simulink model "AFS_VD"  (R2016b)
settings: configuration reference "CodeGenConfigSet" (kept outside this file)
values from neighbouring files (symbols this model uses):
  AFS_dmAirSubsVal_MAP = Calibration.Parameter    [init_AFS_VD.m]
  AFS_dmAirSubsVal_MAPX = Calibration.Parameter    [init_AFS_VD.m]
  AFS_dmAirSubsVal_MAPY = Calibration.Parameter    [init_AFS_VD.m]
  AFS_dtAirThresHi_C = Calibration.Parameter    [init_AFS_VD.m]
  AFS_dtAirThresLo_C = Calibration.Parameter    [init_AFS_VD.m]
  AFS_facAirNrmPT1_C = Calibration.Parameter    [init_AFS_VD.m]
  AFS_facAirSubsEnvPCor_CUR = Calibration.Parameter    [init_AFS_VD.m]
  AFS_facAirSubsEnvPCor_CURX = Calibration.Parameter    [init_AFS_VD.m]
  AFS_facPlsCorBasEGRShOff_MAP = Calibration.Parameter    [init_AFS_VD.m]
  AFS_facPlsCorBasEGRShOff_MAPX = Calibration.Parameter    [init_AFS_VD.m]
  AFS_facPlsCorBasEGRShOff_MAPY = Calibration.Parameter    [init_AFS_VD.m]
  AFS_facPlsCorBasEOMQnt2_MAP = Calibration.Parameter    [init_AFS_VD.m]
  AFS_facPlsCorBasEOMQnt2_MAPX = Calibration.Parameter    [init_AFS_VD.m]
  AFS_facPlsCorBasEOMQnt2_MAPY = Calibration.Parameter    [init_AFS_VD.m]
  AFS_facSwtOnCor_C = Calibration.Parameter    [init_AFS_VD.m]
  AFS_MAIRCONV = int32(33333)    [init_AFS_VD.m]
  AFS_nAvrgThresHi_C = Calibration.Parameter    [init_AFS_VD.m]
  AFS_nAvrgThresLo_C = Calibration.Parameter    [init_AFS_VD.m]
  AFS_numAirTemp_C = Calibration.Parameter    [init_AFS_VD.m]
  AFS_numEngTemp_C = Calibration.Parameter    [init_AFS_VD.m]
  AFS_pAirThrLo_C = Calibration.Parameter    [init_AFS_VD.m]
  AFS_pBstThresHi_C = Calibration.Parameter    [init_AFS_VD.m]
  AFS_pBstThresLo_C = Calibration.Parameter    [init_AFS_VD.m]
  AFS_qRawOvrRunThresHi_C = Calibration.Parameter    [init_AFS_VD.m]
  AFS_qRawOvrRunThresLo_C = Calibration.Parameter    [init_AFS_VD.m]
  AFS_rAirThresIdlHi_C = Calibration.Parameter    [init_AFS_VD.m]
  AFS_rAirThresIdlLo_C = Calibration.Parameter    [init_AFS_VD.m]
  AFS_rAirThresLdHi_C = Calibration.Parameter    [init_AFS_VD.m]
  AFS_rAirThresLdLo_C = Calibration.Parameter    [init_AFS_VD.m]
  AFS_rAirThresOvrRunHi_C = Calibration.Parameter    [init_AFS_VD.m]
  AFS_rAirThresOvrRunLo_C = Calibration.Parameter    [init_AFS_VD.m]
  AFS_rEGRThresHi_C = Calibration.Parameter    [init_AFS_VD.m]
  AFS_rEGRThresLo_C = Calibration.Parameter    [init_AFS_VD.m]
  AFS_rTVAThrHi_C = Calibration.Parameter    [init_AFS_VD.m]
  AFS_rTVAThrLo_C = Calibration.Parameter    [init_AFS_VD.m]
  AFS_swtEnaPlsCor_C = Calibration.Parameter    [init_AFS_VD.m]
  AFS_swtPlausChkIdl_C = Calibration.Parameter    [init_AFS_VD.m]
  AFS_swtPlausChkLd_C = Calibration.Parameter    [init_AFS_VD.m]
  AFS_swtPlausChkOvrRun_C = Calibration.Parameter    [init_AFS_VD.m]
  AFS_swtSensInstVal_C = Calibration.Parameter    [init_AFS_VD.m]
  AFS_tAirThresHi_C = Calibration.Parameter    [init_AFS_VD.m]
  AFS_tAirThresLo_C = Calibration.Parameter    [init_AFS_VD.m]
  AFS_tEngThresHi_C = Calibration.Parameter    [init_AFS_VD.m]
  AFS_tEngThresLo_C = Calibration.Parameter    [init_AFS_VD.m]
  AFS_tiDlyEGRPPlSetyDrft_C = Calibration.Parameter    [init_AFS_VD.m]
  AFS_tiDlySwtOnCor_C = Calibration.Parameter    [init_AFS_VD.m]
  AFS_tiSetyDrftMaxDebDef_C = Calibration.Parameter    [init_AFS_VD.m]
  AFS_tiSetyDrftMaxDebOk_C = Calibration.Parameter    [init_AFS_VD.m]
  AFS_tiSetyDrftMinDebDef_C = Calibration.Parameter    [init_AFS_VD.m]
  AFS_tiSetyDrftMinDebOk_C = Calibration.Parameter    [init_AFS_VD.m]
  Epm_numCyl_C = Calibration.Parameter    [init_AFS_VD.m]
  SigTst_dmAFSVal_C = Calibration.Parameter    [init_AFS_VD.m]
  SigTst_mAirPerCyl_C = Calibration.Parameter    [init_AFS_VD.m]
  SigTst_swtAFSSubsVal_C = Calibration.Parameter    [init_AFS_VD.m]
  SigTst_swtAFSVal_C = Calibration.Parameter    [init_AFS_VD.m]
  SigTst_swtAirPerCyl_C = Calibration.Parameter    [init_AFS_VD.m]
undefined symbols (not defined in the file or in its folder): AFS_VD_DT, EngState_conv, Switch_conv
libraries: simulink x44, CXLib x10
settings Model: Creator=lenovo  LastModifiedBy=guanxiaoxing
settings ConfigSetRef: SourceLocation=Base Workspace

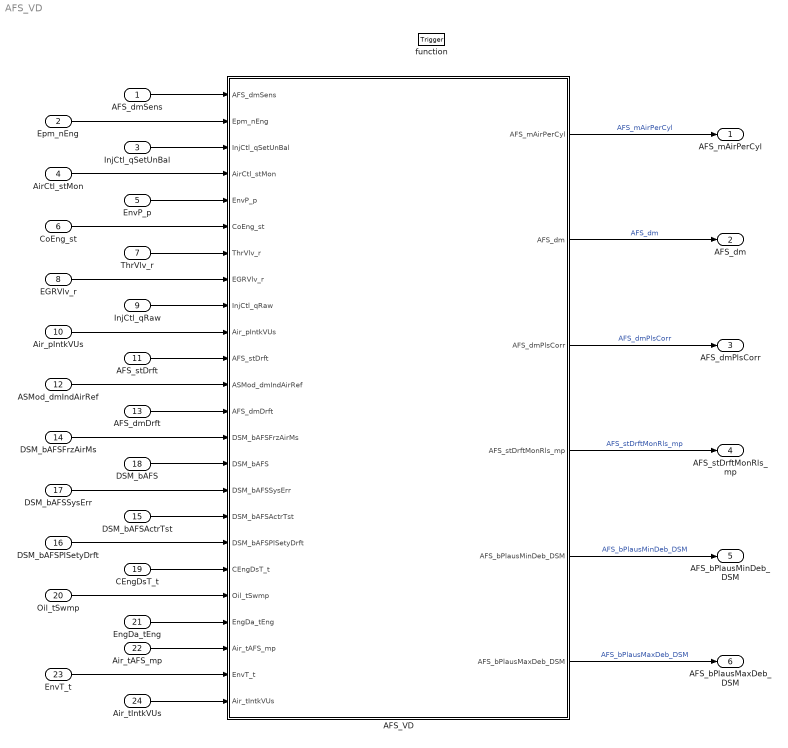
== system AFS_VD ==
  AFS_dmSens : Inport  Tag=kg/h  Description=Processed air mass flow signal of the HFM sensor  OutMin=-8192  OutMax=8191  OutDataTypeStr=AirMassPerTime
  Epm_nEng : Inport  Tag=rpm  Description=Engine speed  Port=2  OutMin=0  OutMax=6000  OutDataTypeStr=EngSpeed_rpm
  InjCtl_qSetUnBal : Inport  Tag=mg/hub  Description=Current injection quantity  Port=3  OutMin=-319  OutMax=319  OutDataTypeStr=FuelMass_mg_hub
  AirCtl_stMon : Inport  Description=status: shutdown case of the governor  Port=4  OutMin=0  OutMax=255  OutDataTypeStr=State_uint8
  EnvP_p : Inport  Tag=kPa  Description=Barometric pressure  Port=5  OutMin=0  OutMax=3276  OutDataTypeStr=AirPressure_kPa
  CoEng_st : Inport  Description=Engine coordinator state  Port=6  OutDataTypeStr=Enum: EngState_conv
  ThrVlv_r : Inport  Tag=%  Description=Commanded value from application SW  Port=7  OutMin=-100  OutMax=100  OutDataTypeStr=Prc_100_rate
  EGRVlv_r : Inport  Tag=%  Description=Commanded value from application SW  Port=8  OutMin=-100  OutMax=100  OutDataTypeStr=Prc_100_rate
  InjCtl_qRaw : Inport  Tag=mg/hub  Description=Raw value of injection mass  Port=9  OutMin=-319  OutMax=319  OutDataTypeStr=FuelMass_mg_hub
  Air_pIntkVUs : Inport  Tag=kPa  Description=Intake valve upstream pressure  Port=10  OutMin=0  OutMax=1200  OutDataTypeStr=AirPressure_kPa
  AFS_stDrft : Inport  Description=Status of drift compensation  Port=11  OutMin=0  OutMax=255  OutDataTypeStr=State_uint8
  ASMod_dmIndAirRef : Inport  Tag=kg/h  Description=Reference of gas mass flow into the engine while exhaust-gas recirculation is closed  Port=12  OutMin=-8192  OutMax=8191  OutDataTypeStr=AirMassPerTime
  AFS_dmDrft : Inport  Tag=kg/h  Description=Compensated Air mass value for the drift  Port=13  OutMin=-8192  OutMax=8191  OutDataTypeStr=AirMassPerTime
  DSM_bAFSFrzAirMs : Inport  Description=Function identifier to freeze the air mass value in case of temporary SRC errors  Port=14  OutMin=0  OutMax=1  OutDataTypeStr=boolean
  DSM_bAFSActrTst : Inport  Description=Function identifier to inhibit checks if remote tester is active for any of the actuators for swirl valve,throttle valve, turbo charger, EGR valve  Port=15  OutMin=0  OutMax=1  OutDataTypeStr=boolean
  DSM_bAFSPlSetyDrft : Inport  Description=Function identifier to inhibit the sensitivity drift check  Port=16  OutMin=0  OutMax=1  OutDataTypeStr=boolean
  DSM_bAFSSysErr : Inport  Description=Function identifier to inhibit the sensitivity drift check  Port=17  OutMin=0  OutMax=1  OutDataTypeStr=boolean
  DSM_bAFS : Inport  Description=Function identifier for switch-over value calculation  Port=18  OutMin=0  OutMax=1  OutDataTypeStr=boolean
  CEngDsT_t : Inport  Tag=deg  Description=engine coolant temperature after filter  Port=19  OutMin=-200  OutMax=200  OutDataTypeStr=Temp_deg
  Oil_tSwmp : Inport  Tag=deg  Description=Oil temperature in oil sump  Port=20  OutMin=-50  OutMax=200  OutDataTypeStr=Temp_deg
  EngDa_tEng : Inport  Tag=deg  Description=Engine temperature  Port=21  OutMin=-1000  OutMax=1000  OutDataTypeStr=Temp_deg
  Air_tAFS_mp : Inport  Tag=deg  Description=Induction air temperature at the HFM  Port=22  OutMin=-200  OutMax=200  OutDataTypeStr=Temp_deg
  EnvT_t : Inport  Tag=deg  Description=Environmental temperature  Port=23  OutMin=-200  OutMax=200  OutDataTypeStr=Temp_deg
  Air_tIntkVUs : Inport  Tag=deg  Description=Intake air temperature upstream of the inlet valve  Port=24  OutMin=-200  OutMax=200  OutDataTypeStr=Temp_deg
  function : TriggerPort  TriggerType=function-call  VariantControl=Variant
  AFS_VD : Subsystem
  AFS_mAirPerCyl : Outport  Tag=mg/hub  Description=Air mass per cylinder  OutMin=0  OutMax=16383  OutDataTypeStr=AirMass_mg_hub
  AFS_dm : Outport  Tag=kg/h  Description=Total air mass flow into the engine  Port=2  OutMin=-8192  OutMax=8191  OutDataTypeStr=AirMassPerTime
  AFS_dmPlsCorr : Outport  Tag=kg/h  Description=Pulsation corrected air mass.  Port=3  OutMin=-8192  OutMax=8191  OutDataTypeStr=AirMassPerTime
  AFS_stDrftMonRls_mp : Outport  Description=Status of monitoring conditions for the sensitivity drift test  Port=4  OutMin=0  OutMax=1  OutDataTypeStr=boolean
  AFS_bPlausMinDeb_DSM : Outport  Description=fault flag for plausibility check of Min error  Port=5  OutMin=0  OutMax=1  OutDataTypeStr=boolean
  AFS_bPlausMaxDeb_DSM : Outport  Description=fault flag for plausibility check of Max error  Port=6  OutMin=0  OutMax=1  OutDataTypeStr=boolean
  wires:
  AFS_VD/1(AFS_mAirPerCyl) -> AFS_mAirPerCyl/1  "AFS_mAirPerCyl"
  AFS_VD/2(AFS_dm) -> AFS_dm/1  "AFS_dm"
  AFS_VD/3(AFS_dmPlsCorr) -> AFS_dmPlsCorr/1  "AFS_dmPlsCorr"
  AFS_VD/4(AFS_stDrftMonRls_mp) -> AFS_stDrftMonRls_mp/1  "AFS_stDrftMonRls_mp"
  AFS_VD/5(AFS_bPlausMinDeb_DSM) -> AFS_bPlausMinDeb_DSM/1  "AFS_bPlausMinDeb_DSM"
  AFS_VD/6(AFS_bPlausMaxDeb_DSM) -> AFS_bPlausMaxDeb_DSM/1  "AFS_bPlausMaxDeb_DSM"
  AFS_dmSens/1 -> AFS_VD/1(AFS_dmSens)
  Epm_nEng/1 -> AFS_VD/2(Epm_nEng)
  InjCtl_qSetUnBal/1 -> AFS_VD/3(InjCtl_qSetUnBal)
  AirCtl_stMon/1 -> AFS_VD/4(AirCtl_stMon)
  EnvP_p/1 -> AFS_VD/5(EnvP_p)
  CoEng_st/1 -> AFS_VD/6(CoEng_st)
  ThrVlv_r/1 -> AFS_VD/7(ThrVlv_r)
  EGRVlv_r/1 -> AFS_VD/8(EGRVlv_r)
  InjCtl_qRaw/1 -> AFS_VD/9(InjCtl_qRaw)
  Air_pIntkVUs/1 -> AFS_VD/10(Air_pIntkVUs)
  AFS_stDrft/1 -> AFS_VD/11(AFS_stDrft)
  ASMod_dmIndAirRef/1 -> AFS_VD/12(ASMod_dmIndAirRef)
  AFS_dmDrft/1 -> AFS_VD/13(AFS_dmDrft)
  DSM_bAFSFrzAirMs/1 -> AFS_VD/14(DSM_bAFSFrzAirMs)
  DSM_bAFS/1 -> AFS_VD/15(DSM_bAFS)
  DSM_bAFSActrTst/1 -> AFS_VD/17(DSM_bAFSActrTst)
  DSM_bAFSSysErr/1 -> AFS_VD/16(DSM_bAFSSysErr)
  DSM_bAFSPlSetyDrft/1 -> AFS_VD/18(DSM_bAFSPlSetyDrft)
  CEngDsT_t/1 -> AFS_VD/19(CEngDsT_t)
  Oil_tSwmp/1 -> AFS_VD/20(Oil_tSwmp)
  EngDa_tEng/1 -> AFS_VD/21(EngDa_tEng)
  Air_tAFS_mp/1 -> AFS_VD/22(Air_tAFS_mp)
  EnvT_t/1 -> AFS_VD/23(EnvT_t)
  Air_tIntkVUs/1 -> AFS_VD/24(Air_tIntkVUs)

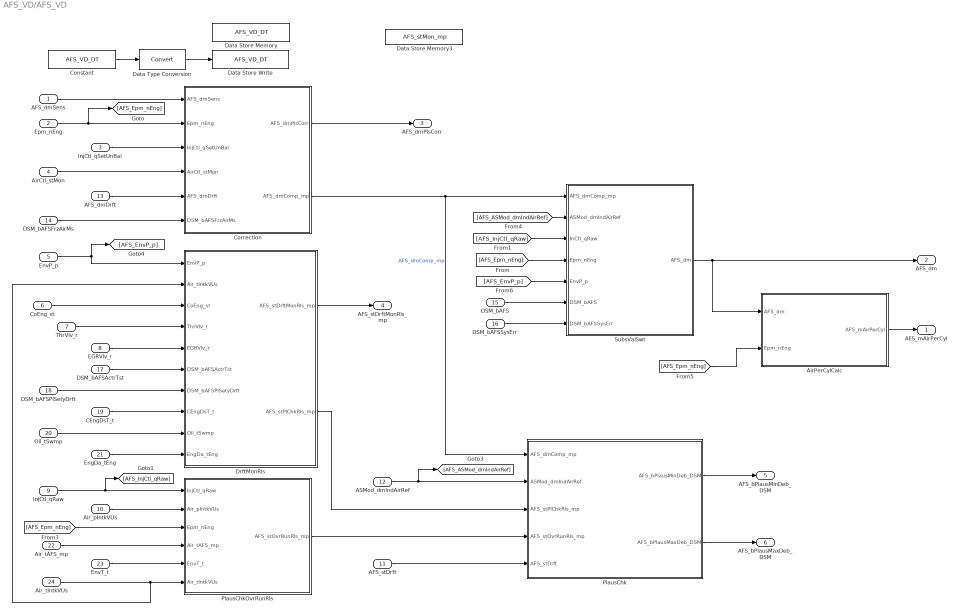
== system AFS_VD/AFS_VD ==
  AFS_dmSens : Inport
  Epm_nEng : Inport  Port=2
  InjCtl_qSetUnBal : Inport  Port=3
  AirCtl_stMon : Inport  Port=4
  EnvP_p : Inport  Port=5
  CoEng_st : Inport  Port=6
  ThrVlv_r : Inport  Port=7
  EGRVlv_r : Inport  Port=8
  InjCtl_qRaw : Inport  Port=9
  Air_pIntkVUs : Inport  Port=10
  AFS_stDrft : Inport  Port=11
  ASMod_dmIndAirRef : Inport  Port=12
  AFS_dmDrft : Inport  Port=13
  DSM_bAFSFrzAirMs : Inport  Port=14
  DSM_bAFS : Inport  Port=15
  DSM_bAFSSysErr : Inport  Port=16
  DSM_bAFSActrTst : Inport  Port=17
  DSM_bAFSPlSetyDrft : Inport  Port=18
  CEngDsT_t : Inport  Port=19
  Oil_tSwmp : Inport  Port=20
  EngDa_tEng : Inport  Port=21
  Air_tAFS_mp : Inport  Port=22
  EnvT_t : Inport  Port=23
  Air_tIntkVUs : Inport  Port=24
  AirPerCylCalc : Subsystem
  Constant : Constant  Value=AFS_VD_DT
  Correction : Subsystem
  Data Store Memory : DataStoreMemory  DataStoreName=AFS_VD_DT  ReadBeforeWriteMsg=warning  WriteAfterWriteMsg=warning  WriteAfterReadMsg=warning  ShowAdditionalParam=off
  Data Store Memory3 : DataStoreMemory  DataStoreName=AFS_stMon_mp  ReadBeforeWriteMsg=warning  WriteAfterWriteMsg=warning  WriteAfterReadMsg=warning  ShowAdditionalParam=off  StateMustResolveToSignalObject=on
  Data Store Write : DataStoreWrite  DataStoreName=AFS_VD_DT
  Data Type Conversion : DataTypeConversion
  DrftMonRls : Subsystem
  PlausChk : Subsystem
  PlausChkOvrRunRls : Subsystem
  SubsValSwt : Subsystem
  AFS_mAirPerCyl : Outport
  AFS_dm : Outport  Port=2
  AFS_dmPlsCorr : Outport  Port=3
  AFS_stDrftMonRls_mp : Outport  Port=4
  AFS_bPlausMinDeb_DSM : Outport  Port=5
  AFS_bPlausMaxDeb_DSM : Outport  Port=6
  wires:
  Epm_nEng/1 -> [AFS_Epm_nEng], Correction/2(Epm_nEng)
  InjCtl_qRaw/1 -> PlausChkOvrRunRls/1(InjCtl_qRaw), [AFS_InjCtl_qRaw]
  Air_pIntkVUs/1 -> PlausChkOvrRunRls/2(Air_pIntkVUs)
  DrftMonRls/2(AFS_stPlChkRls_mp) -> PlausChk/3(AFS_stPlChkRls_mp)
  DrftMonRls/1(AFS_stDrftMonRls_mp) -> AFS_stDrftMonRls_mp/1
  AirPerCylCalc/1(AFS_mAirPerCyl) -> AFS_mAirPerCyl/1
  [AFS_Epm_nEng] -> AirPerCylCalc/2(Epm_nEng)
  Air_tIntkVUs/1 -> DrftMonRls/2(Air_tIntkVUs), PlausChkOvrRunRls/6(Air_tIntkVUs)
  CoEng_st/1 -> DrftMonRls/3(CoEng_st)
  ThrVlv_r/1 -> DrftMonRls/4(ThrVlv_r)
  EGRVlv_r/1 -> DrftMonRls/5(EGRVlv_r)
  AFS_stDrft/1 -> PlausChk/5(AFS_stDrft)
  ASMod_dmIndAirRef/1 -> PlausChk/2(ASMod_dmIndAirRef), [AFS_ASMod_dmIndAirRef]
  PlausChkOvrRunRls/1(AFS_stOvrRunRls_mp) -> PlausChk/4(AFS_stOvrRunRls_mp)
  [AFS_Epm_nEng] -> PlausChkOvrRunRls/3(Epm_nEng)
  SubsValSwt/1(AFS_dm) -> AFS_dm/1, AirPerCylCalc/1(AFS_dm)
  EnvP_p/1 -> [AFS_EnvP_p], DrftMonRls/1(EnvP_p)
  [AFS_InjCtl_qRaw] -> SubsValSwt/3(InCtl_qRaw)
  [AFS_Epm_nEng] -> SubsValSwt/4(Epm_nEng)
  [AFS_ASMod_dmIndAirRef] -> SubsValSwt/2(ASMod_dmIndAirRef)
  [AFS_EnvP_p] -> SubsValSwt/5(EnvP_p)
  Constant/1 -> Data Type Conversion/1
  Correction/2(AFS_dmComp_mp) -> SubsValSwt/1(AFS_dmComp_mp), PlausChk/1(AFS_dmComp_mp)  "AFS_dmComp_mp"
  AFS_dmSens/1 -> Correction/1(AFS_dmSens)
  InjCtl_qSetUnBal/1 -> Correction/3(InjCtl_qSetUnBal)
  AirCtl_stMon/1 -> Correction/4(AirCtl_stMon)
  AFS_dmDrft/1 -> Correction/5(AFS_dmDrft)
  DSM_bAFSFrzAirMs/1 -> Correction/6(DSM_bAFSFrzAirMs)
  Correction/1(AFS_dmPlsCorr) -> AFS_dmPlsCorr/1
  DSM_bAFS/1 -> SubsValSwt/6(DSM_bAFS)
  DSM_bAFSSysErr/1 -> SubsValSwt/7(DSM_bAFSSysErr)
  DSM_bAFSActrTst/1 -> DrftMonRls/6(DSM_bAFSActrTst)
  DSM_bAFSPlSetyDrft/1 -> DrftMonRls/7(DSM_bAFSPlSetyDrft)
  CEngDsT_t/1 -> DrftMonRls/8(CEngDsT_t)
  Oil_tSwmp/1 -> DrftMonRls/9(Oil_tSwmp)
  EngDa_tEng/1 -> DrftMonRls/10(EngDa_tEng)
  Air_tAFS_mp/1 -> PlausChkOvrRunRls/4(Air_tAFS_mp)
  EnvT_t/1 -> PlausChkOvrRunRls/5(EnvT_t)
  PlausChk/1(AFS_bPlausMinDeb_DSM) -> AFS_bPlausMinDeb_DSM/1
  PlausChk/2(AFS_bPlausMaxDeb_DSM) -> AFS_bPlausMaxDeb_DSM/1
  Data Type Conversion/1 -> Data Store Write/1

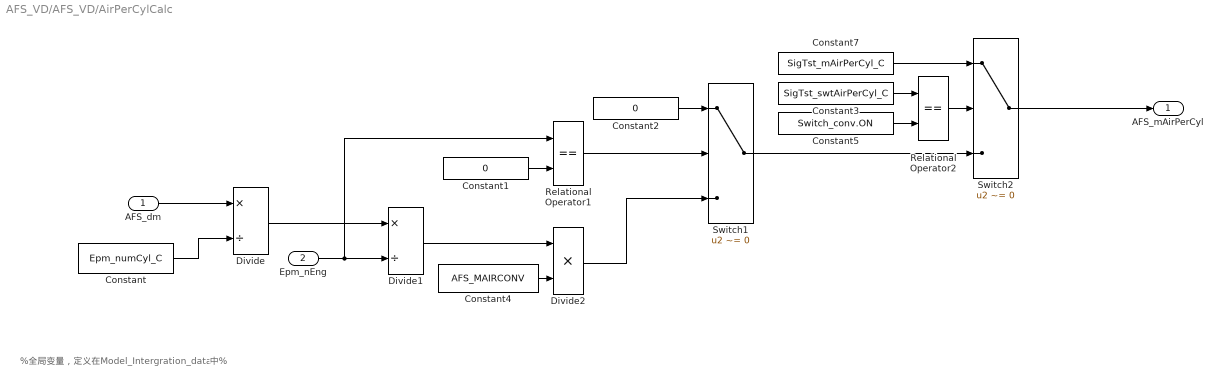
== system AFS_VD/AFS_VD/AirPerCylCalc ==
  note: %全局变量，定义在Model_Intergration_data中%
  AFS_dm : Inport
  Epm_nEng : Inport  Port=2
  Constant : Constant  Value=Epm_numCyl_C
  Constant1 : Constant  Value=0  OutDataTypeStr=EngSpeed_rpm
  Constant2 : Constant  Value=0  OutDataTypeStr=AirMass_mg_hub
  Constant3 : Constant  Value=SigTst_swtAirPerCyl_C
  Constant4 : Constant  Value=AFS_MAIRCONV
  Constant5 : Constant  Value=Switch_conv.ON
  Constant7 : Constant  Value=SigTst_mAirPerCyl_C
  Divide : Product  Inputs=*/  OutDataTypeStr=Inherit: Inherit via back propagation  SaturateOnIntegerOverflow=on
  Divide1 : Product  Inputs=*/  OutDataTypeStr=fixdt(1,32,16)  SaturateOnIntegerOverflow=on
  Divide2 : Product  Inputs=**  OutDataTypeStr=Inherit: Inherit via back propagation  SaturateOnIntegerOverflow=on
  Relational Operator1 : RelationalOperator  Operator===  OutDataTypeStr=boolean  RndMeth=Nearest  InputSameDT=on
  Relational Operator2 : RelationalOperator  Operator===  OutDataTypeStr=boolean  RndMeth=Nearest  InputSameDT=on
  Switch1 : Switch  Criteria=u2 ~= 0  OutDataTypeStr=Inherit: Inherit via back propagation  SaturateOnIntegerOverflow=on  InputSameDT=on
  Switch2 : Switch  Criteria=u2 ~= 0  OutDataTypeStr=Inherit: Inherit via back propagation  SaturateOnIntegerOverflow=on  InputSameDT=on
  AFS_mAirPerCyl : Outport
  wires:
  Constant5/1 -> Relational Operator2/2
  Switch1/1 -> Switch2/3
  Constant7/1 -> Switch2/1
  Relational Operator2/1 -> Switch2/2
  Constant3/1 -> Relational Operator2/1
  Constant2/1 -> Switch1/1
  Divide2/1 -> Switch1/3
  AFS_dm/1 -> Divide/1
  Relational Operator1/1 -> Switch1/2
  Constant1/1 -> Relational Operator1/2
  Epm_nEng/1 -> Divide1/2, Relational Operator1/1
  Constant4/1 -> Divide2/2
  Divide/1 -> Divide1/1
  Divide1/1 -> Divide2/1
  Switch2/1 -> AFS_mAirPerCyl/1
  Constant/1 -> Divide/2

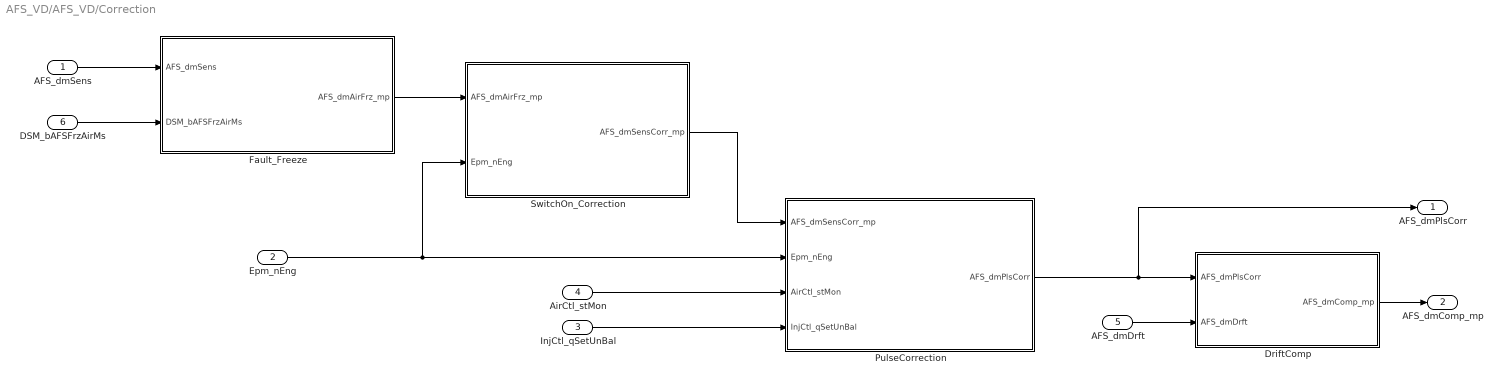
== system AFS_VD/AFS_VD/Correction ==
  AFS_dmSens : Inport
  Epm_nEng : Inport  Port=2
  InjCtl_qSetUnBal : Inport  Port=3
  AirCtl_stMon : Inport  Port=4
  AFS_dmDrft : Inport  Port=5
  DSM_bAFSFrzAirMs : Inport  Port=6
  DriftComp : Subsystem
  Fault_Freeze : Subsystem
  PulseCorrection : Subsystem
  SwitchOn_Correction : Subsystem
  AFS_dmPlsCorr : Outport
  AFS_dmComp_mp : Outport  Port=2
  wires:
  PulseCorrection/1(AFS_dmPlsCorr) -> DriftComp/1(AFS_dmPlsCorr), AFS_dmPlsCorr/1
  InjCtl_qSetUnBal/1 -> PulseCorrection/4(InjCtl_qSetUnBal)
  AirCtl_stMon/1 -> PulseCorrection/3(AirCtl_stMon)
  SwitchOn_Correction/1(AFS_dmSensCorr_mp) -> PulseCorrection/1(AFS_dmSensCorr_mp)
  Fault_Freeze/1(AFS_dmAirFrz_mp) -> SwitchOn_Correction/1(AFS_dmAirFrz_mp)
  Epm_nEng/1 -> SwitchOn_Correction/2(Epm_nEng), PulseCorrection/2(Epm_nEng)
  AFS_dmSens/1 -> Fault_Freeze/1(AFS_dmSens)
  DSM_bAFSFrzAirMs/1 -> Fault_Freeze/2(DSM_bAFSFrzAirMs)
  AFS_dmDrft/1 -> DriftComp/2(AFS_dmDrft)
  DriftComp/1(AFS_dmComp_mp) -> AFS_dmComp_mp/1

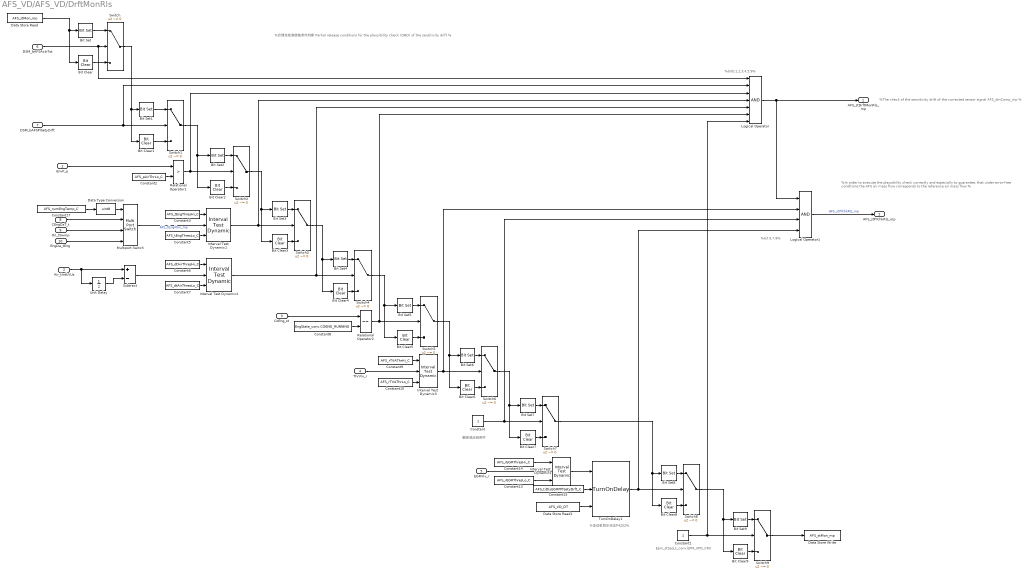
== system AFS_VD/AFS_VD/DrftMonRls ==
  note: Epm_stSpd_t_conv.EPM_SPD_CRS
  note: 删掉涡流阀条件
  note: %发动机同步状态P4252%
  note: %bit0,1,2,3,4,5,9%
  note: %bit 6,7,8%
  note: %The check of the sensitivity drift of the corrected sensor signal AFS_dmComp_mp %
  note: %In order to execute the plausibility check correctly and especially to guarantee, that under error-free conditions the AFS air mass flow corresponds
      | to the reference air mass flow %
  note: %合理性检测使能条件判断
      | Partial release conditions for the plausibility check (OBD) of the sensitivity drift %
  EnvP_p : Inport
  Air_tIntkVUs : Inport  Port=2
  CoEng_st : Inport  Port=3
  ThrVlv_r : Inport  Port=4
  EGRVlv_r : Inport  Port=5
  DSM_bAFSActrTst : Inport  Port=6
  DSM_bAFSPlSetyDrft : Inport  Port=7
  CEngDsT_t : Inport  Port=8
  Oil_tSwmp : Inport  Port=9
  EngDa_tEng : Inport  Port=10
  Bit Clear : simulink/Logic and Bit Operations/Bit Clear  iBit=0
  Bit Clear1 : simulink/Logic and Bit Operations/Bit Clear  iBit=1
  Bit Clear2 : simulink/Logic and Bit Operations/Bit Clear  iBit=2
  Bit Clear3 : simulink/Logic and Bit Operations/Bit Clear  iBit=3
  Bit Clear4 : simulink/Logic and Bit Operations/Bit Clear  iBit=4
  Bit Clear5 : simulink/Logic and Bit Operations/Bit Clear  iBit=5
  Bit Clear6 : simulink/Logic and Bit Operations/Bit Clear  iBit=6
  Bit Clear7 : simulink/Logic and Bit Operations/Bit Clear  iBit=7
  Bit Clear8 : simulink/Logic and Bit Operations/Bit Clear  iBit=8
  Bit Clear9 : simulink/Logic and Bit Operations/Bit Clear  iBit=9
  Bit Set : simulink/Logic and Bit Operations/Bit Set  iBit=0
  Bit Set1 : simulink/Logic and Bit Operations/Bit Set  iBit=1
  Bit Set2 : simulink/Logic and Bit Operations/Bit Set  iBit=2
  Bit Set3 : simulink/Logic and Bit Operations/Bit Set  iBit=3
  Bit Set4 : simulink/Logic and Bit Operations/Bit Set  iBit=4
  Bit Set5 : simulink/Logic and Bit Operations/Bit Set  iBit=5
  Bit Set6 : simulink/Logic and Bit Operations/Bit Set  iBit=6
  Bit Set7 : simulink/Logic and Bit Operations/Bit Set  iBit=7
  Bit Set8 : simulink/Logic and Bit Operations/Bit Set  iBit=8
  Bit Set9 : simulink/Logic and Bit Operations/Bit Set  iBit=9
  Constant : Constant  OutDataTypeStr=boolean
  Constant1 : Constant  OutDataTypeStr=boolean
  Constant10 : Constant  Value=AFS_rTVAThrLo_C
  Constant13 : Constant  Value=AFS_rEGRThresLo_C
  Constant14 : Constant  Value=AFS_rEGRThresHi_C
  Constant15 : Constant  Value=AFS_tiDlyEGRPPlSetyDrft_C
  Constant17 : Constant  Value=AFS_numEngTemp_C
  Constant2 : Constant  Value=AFS_pAirThrLo_C
  Constant3 : Constant  Value=AFS_tEngThresHi_C
  Constant5 : Constant  Value=AFS_tEngThresLo_C
  Constant6 : Constant  Value=AFS_dtAirThresHi_C
  Constant7 : Constant  Value=AFS_dtAirThresLo_C
  Constant8 : Constant  Value=EngState_conv.COENG_RUNNING
  Constant9 : Constant  Value=AFS_rTVAThrHi_C
  Data Store Read : DataStoreRead  DataStoreName=AFS_stMon_mp
  Data Store Read1 : DataStoreRead  DataStoreName=AFS_VD_DT
  Data Store Write : DataStoreWrite  DataStoreName=AFS_stMon_mp
  Data Type Conversion : DataTypeConversion  OutDataTypeStr=uint8
  Interval Test Dynamic{1..3,5} (4 alike) : simulink/Logic and Bit Operations/Interval Test Dynamic  IntervalClosedRight=on  IntervalClosedLeft=on  OutDataTypeStr=boolean
  Logical Operator : Logic  Inputs=7  AllPortsSameDT=off  OutDataTypeStr=boolean
  Logical Operator1 : Logic  Inputs=4  AllPortsSameDT=off  OutDataTypeStr=boolean
  Multiport Switch : MultiPortSwitch  DataPortOrder=Zero-based contiguous
  Relational Operator1 : RelationalOperator  Operator=>  OutDataTypeStr=boolean  RndMeth=Nearest  InputSameDT=on
  Relational Operator2 : RelationalOperator  Operator===  OutDataTypeStr=boolean  RndMeth=Nearest  InputSameDT=on
  Subtract : Sum  Inputs=+-  OutDataTypeStr=Temp_deg_s
  Switch{,1..9} (10 alike) : Switch  Criteria=u2 ~= 0  OutDataTypeStr=Inherit: Inherit via back propagation  SaturateOnIntegerOverflow=on  InputSameDT=on
  TurnOnDelay1 : CXLib/TurnOnDelay
  Unit Delay : UnitDelay  SampleTime=-1
  AFS_stDrftMonRls_mp : Outport
  AFS_stPlChkRls_mp : Outport  Port=2
  wires:
  Multiport Switch/1 -> Interval Test Dynamic1/2  "AFS_tEngMon_mp"
  Constant17/1 -> Data Type Conversion/1
  Switch9/1 -> Data Store Write/1
  TurnOnDelay1/1 -> Logical Operator1/4, Switch8/2
  Interval Test Dynamic5/1 -> TurnOnDelay1/1
  Constant15/1 -> TurnOnDelay1/2
  Switch7/1 -> Bit Set8/1, Bit Clear8/1
  Data Store Read1/1 -> TurnOnDelay1/3
  Bit Clear8/1 -> Switch8/3
  Constant13/1 -> Interval Test Dynamic5/3
  Constant14/1 -> Interval Test Dynamic5/1
  EGRVlv_r/1 -> Interval Test Dynamic5/2
  Bit Set8/1 -> Switch8/1
  Interval Test Dynamic3/1 -> Switch6/2, Logical Operator1/2
  Switch6/1 -> Bit Clear7/1, Bit Set7/1
  Bit Set7/1 -> Switch7/1
  Constant10/1 -> Interval Test Dynamic3/3
  Constant9/1 -> Interval Test Dynamic3/1
  Bit Clear7/1 -> Switch7/3
  Bit Set6/1 -> Switch6/1
  Bit Clear6/1 -> Switch6/3
  Bit Set5/1 -> Switch5/1
  Switch5/1 -> Bit Set6/1, Bit Clear6/1
  ThrVlv_r/1 -> Interval Test Dynamic3/2
  Switch1/1 -> Bit Set2/1, Bit Clear2/1
  Constant3/1 -> Interval Test Dynamic1/1
  Relational Operator1/1 -> Switch2/2, Logical Operator/3
  Bit Clear1/1 -> Switch1/3
  Switch2/1 -> Bit Set3/1, Bit Clear3/1
  Bit Set3/1 -> Switch3/1
  Interval Test Dynamic1/1 -> Switch3/2, Logical Operator/4
  Bit Clear3/1 -> Switch3/3
  Switch3/1 -> Bit Clear4/1, Bit Set4/1
  Bit Clear4/1 -> Switch4/3
  Bit Set4/1 -> Switch4/1
  Interval Test Dynamic2/1 -> Switch4/2, Logical Operator/5
  Constant7/1 -> Interval Test Dynamic2/3
  Constant6/1 -> Interval Test Dynamic2/1
  Constant2/1 -> Relational Operator1/2
  Constant5/1 -> Interval Test Dynamic1/3
  Switch4/1 -> Bit Clear5/1, Bit Set5/1
  Constant8/1 -> Relational Operator2/2
  Relational Operator2/1 -> Switch5/2, Logical Operator/6
  Bit Clear5/1 -> Switch5/3
  Switch/1 -> Bit Clear1/1, Bit Set1/1
  CoEng_st/1 -> Relational Operator2/1
  Switch8/1 -> Bit Clear9/1, Bit Set9/1
  Bit Clear9/1 -> Switch9/3
  Bit Set9/1 -> Switch9/1
  Logical Operator1/1 -> AFS_stPlChkRls_mp/1  "AFS_stPlChkRls_mp"
  Logical Operator/1 -> Logical Operator1/1, AFS_stDrftMonRls_mp/1
  Bit Set/1 -> Switch/1
  DSM_bAFSActrTst/1 -> Switch/2, Logical Operator/1
  EnvP_p/1 -> Relational Operator1/1
  Bit Clear/1 -> Switch/3
  Data Store Read/1 -> Bit Clear/1, Bit Set/1
  Bit Set1/1 -> Switch1/1
  DSM_bAFSPlSetyDrft/1 -> Switch1/2, Logical Operator/2
  Bit Clear2/1 -> Switch2/3
  Bit Set2/1 -> Switch2/1
  CEngDsT_t/1 -> Multiport Switch/2
  Oil_tSwmp/1 -> Multiport Switch/3
  EngDa_tEng/1 -> Multiport Switch/4
  Data Type Conversion/1 -> Multiport Switch/1
  Air_tIntkVUs/1 -> Unit Delay/1, Subtract/1
  Subtract/1 -> Interval Test Dynamic2/2
  Unit Delay/1 -> Subtract/2
  Constant/1 -> Logical Operator1/3, Switch7/2
  Constant1/1 -> Logical Operator/7, Switch9/2

== system AFS_VD/AFS_VD/PlausChk ==
  AFS_dmComp_mp : Inport
  ASMod_dmIndAirRef : Inport  Port=2
  AFS_stPlChkRls_mp : Inport  Port=3
  AFS_stOvrRunRls_mp : Inport  Port=4
  AFS_stDrft : Inport  Port=5
  Detect : Subsystem
  Monitor_Fault : Subsystem
  AFS_bPlausMinDeb_DSM : Outport
  AFS_bPlausMaxDeb_DSM : Outport  Port=2
  wires:
  AFS_stDrft/1 -> Detect/1(AFS_stDrft)
  AFS_dmComp_mp/1 -> Detect/2(AFS_dmComp_mp)
  ASMod_dmIndAirRef/1 -> Detect/3(ASMod_dmIndAirRef)
  AFS_stPlChkRls_mp/1 -> Monitor_Fault/1(AFS_stPlChkRls_mp)
  AFS_stOvrRunRls_mp/1 -> Monitor_Fault/2(AFS_stOvrRunRls_mp)
  Detect/1(stLoadRls) -> Monitor_Fault/3(stLoadRls)
  Detect/2(stIdlRls) -> Monitor_Fault/4(stIdlRls)
  Detect/3(stPlausMin) -> Monitor_Fault/5(stPlausMin)
  Detect/4(stPlausMax) -> Monitor_Fault/6(stPlausMax)
  Monitor_Fault/2(AFS_bPlausMaxDeb_DSM) -> AFS_bPlausMaxDeb_DSM/1
  Monitor_Fault/1(AFS_bPlausMinDeb_DSM) -> AFS_bPlausMinDeb_DSM/1

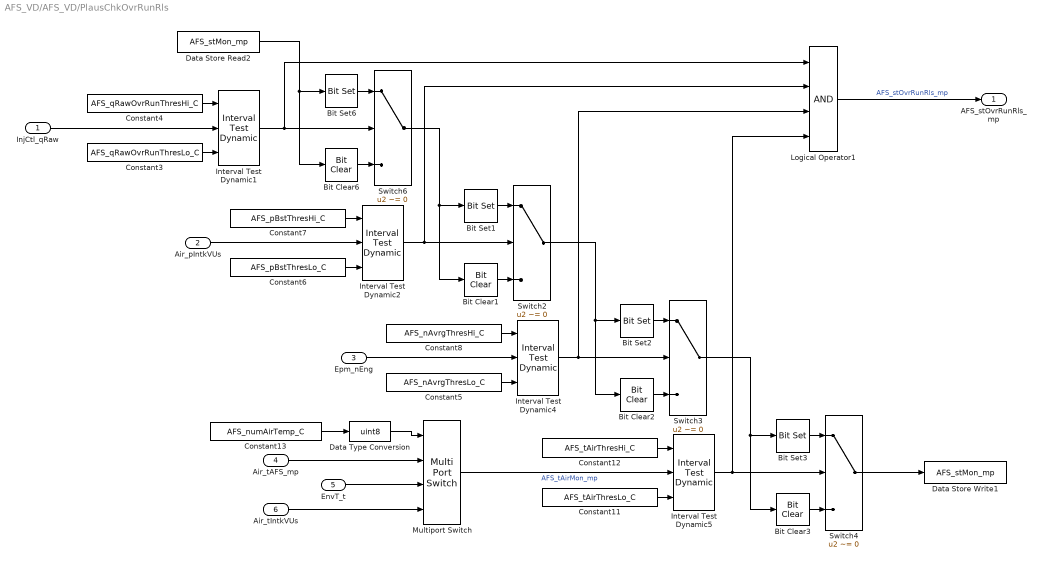
== system AFS_VD/AFS_VD/PlausChkOvrRunRls ==
  InjCtl_qRaw : Inport
  Air_pIntkVUs : Inport  Port=2
  Epm_nEng : Inport  Port=3
  Air_tAFS_mp : Inport  Port=4
  EnvT_t : Inport  Port=5
  Air_tIntkVUs : Inport  Port=6
  Bit Clear1 : simulink/Logic and Bit Operations/Bit Clear  iBit=16
  Bit Clear2 : simulink/Logic and Bit Operations/Bit Clear  iBit=17
  Bit Clear3 : simulink/Logic and Bit Operations/Bit Clear  iBit=18
  Bit Clear6 : simulink/Logic and Bit Operations/Bit Clear  iBit=15
  Bit Set1 : simulink/Logic and Bit Operations/Bit Set  iBit=16
  Bit Set2 : simulink/Logic and Bit Operations/Bit Set  iBit=17
  Bit Set3 : simulink/Logic and Bit Operations/Bit Set  iBit=18
  Bit Set6 : simulink/Logic and Bit Operations/Bit Set  iBit=15
  Constant11 : Constant  Value=AFS_tAirThresLo_C
  Constant12 : Constant  Value=AFS_tAirThresHi_C
  Constant13 : Constant  Value=AFS_numAirTemp_C
  Constant3 : Constant  Value=AFS_qRawOvrRunThresLo_C
  Constant4 : Constant  Value=AFS_qRawOvrRunThresHi_C
  Constant5 : Constant  Value=AFS_nAvrgThresLo_C
  Constant6 : Constant  Value=AFS_pBstThresLo_C
  Constant7 : Constant  Value=AFS_pBstThresHi_C
  Constant8 : Constant  Value=AFS_nAvrgThresHi_C
  Data Store Read2 : DataStoreRead  DataStoreName=AFS_stMon_mp
  Data Store Write1 : DataStoreWrite  DataStoreName=AFS_stMon_mp
  Data Type Conversion : DataTypeConversion  OutDataTypeStr=uint8
  Interval Test Dynamic{1..2,4..5} (4 alike) : simulink/Logic and Bit Operations/Interval Test Dynamic  IntervalClosedRight=on  IntervalClosedLeft=on  OutDataTypeStr=boolean
  Logical Operator1 : Logic  Inputs=4  AllPortsSameDT=off  OutDataTypeStr=boolean
  Multiport Switch : MultiPortSwitch  DataPortOrder=Zero-based contiguous
  Switch{2..4,6} (4 alike) : Switch  Criteria=u2 ~= 0  OutDataTypeStr=Inherit: Inherit via back propagation  SaturateOnIntegerOverflow=on  InputSameDT=on
  AFS_stOvrRunRls_mp : Outport
  wires:
  Multiport Switch/1 -> Interval Test Dynamic5/2  "AFS_tAirMon_mp"
  Constant13/1 -> Data Type Conversion/1
  Logical Operator1/1 -> AFS_stOvrRunRls_mp/1  "AFS_stOvrRunRls_mp"
  Switch4/1 -> Data Store Write1/1
  Constant11/1 -> Interval Test Dynamic5/3
  Constant12/1 -> Interval Test Dynamic5/1
  Switch3/1 -> Bit Clear3/1, Bit Set3/1
  Bit Set3/1 -> Switch4/1
  Interval Test Dynamic5/1 -> Switch4/2, Logical Operator1/4
  Bit Clear3/1 -> Switch4/3
  Constant5/1 -> Interval Test Dynamic4/3
  Constant8/1 -> Interval Test Dynamic4/1
  Epm_nEng/1 -> Interval Test Dynamic4/2
  Switch2/1 -> Bit Set2/1, Bit Clear2/1
  Bit Set2/1 -> Switch3/1
  Interval Test Dynamic4/1 -> Switch3/2, Logical Operator1/3
  Bit Clear2/1 -> Switch3/3
  Interval Test Dynamic1/1 -> Switch6/2, Logical Operator1/1
  Constant6/1 -> Interval Test Dynamic2/3
  Constant7/1 -> Interval Test Dynamic2/1
  Air_pIntkVUs/1 -> Interval Test Dynamic2/2
  Constant3/1 -> Interval Test Dynamic1/3
  Constant4/1 -> Interval Test Dynamic1/1
  InjCtl_qRaw/1 -> Interval Test Dynamic1/2
  Bit Set6/1 -> Switch6/1
  Bit Clear6/1 -> Switch6/3
  Data Store Read2/1 -> Bit Set6/1, Bit Clear6/1
  Switch6/1 -> Bit Clear1/1, Bit Set1/1
  Bit Set1/1 -> Switch2/1
  Interval Test Dynamic2/1 -> Switch2/2, Logical Operator1/2
  Bit Clear1/1 -> Switch2/3
  Data Type Conversion/1 -> Multiport Switch/1
  Air_tIntkVUs/1 -> Multiport Switch/4
  Air_tAFS_mp/1 -> Multiport Switch/2
  EnvT_t/1 -> Multiport Switch/3

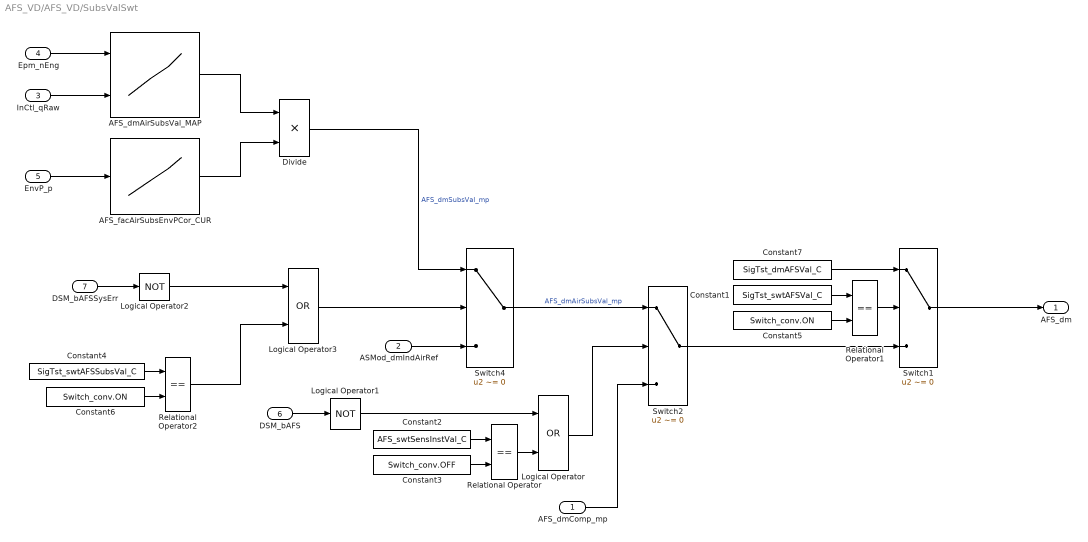
== system AFS_VD/AFS_VD/SubsValSwt ==
  AFS_dmComp_mp : Inport
  ASMod_dmIndAirRef : Inport  Port=2
  InCtl_qRaw : Inport  Port=3
  Epm_nEng : Inport  Port=4
  EnvP_p : Inport  Port=5
  DSM_bAFS : Inport  Port=6
  DSM_bAFSSysErr : Inport  Port=7
  AFS_dmAirSubsVal_MAP : Lookup_n-D  BreakpointsForDimension1=AFS_dmAirSubsVal_MAPY  BreakpointsForDimension2=AFS_dmAirSubsVal_MAPX  IndexSearchMethod=Linear search  BeginIndexSearchUsingPreviousIndexResult=on  Table=AFS_dmAirSubsVal_MAP  ExtrapMethod=Clip  UseLastTableValue=on  InternalRulePriority=Speed  OutDataTypeStr=Inherit: Inherit via back propagation  SaturateOnIntegerOverflow=on
  AFS_facAirSubsEnvPCor_CUR : Lookup_n-D  NumberOfTableDimensions=1  BreakpointsForDimension1=AFS_facAirSubsEnvPCor_CURX  IndexSearchMethod=Linear search  BeginIndexSearchUsingPreviousIndexResult=on  UseOneInputPortForAllInputData=on  Table=AFS_facAirSubsEnvPCor_CUR  ExtrapMethod=Clip  UseLastTableValue=on  InternalRulePriority=Speed  OutDataTypeStr=Inherit: Inherit via back propagation  SaturateOnIntegerOverflow=on
  Constant1 : Constant  Value=SigTst_swtAFSVal_C
  Constant2 : Constant  Value=AFS_swtSensInstVal_C
  Constant3 : Constant  Value=Switch_conv.OFF
  Constant4 : Constant  Value=SigTst_swtAFSSubsVal_C
  Constant5 : Constant  Value=Switch_conv.ON
  Constant6 : Constant  Value=Switch_conv.ON
  Constant7 : Constant  Value=SigTst_dmAFSVal_C
  Divide : Product  Inputs=**  OutDataTypeStr=Inherit: Inherit via back propagation  SaturateOnIntegerOverflow=on
  Logical Operator : Logic  Operator=OR  AllPortsSameDT=off  OutDataTypeStr=boolean
  Logical Operator1 : Logic  Operator=NOT  AllPortsSameDT=off  OutDataTypeStr=boolean
  Logical Operator2 : Logic  Operator=NOT  AllPortsSameDT=off  OutDataTypeStr=boolean
  Logical Operator3 : Logic  Operator=OR  AllPortsSameDT=off  OutDataTypeStr=boolean
  Relational Operator : RelationalOperator  Operator===  OutDataTypeStr=boolean  RndMeth=Nearest  InputSameDT=on
  Relational Operator1 : RelationalOperator  Operator===  OutDataTypeStr=boolean  RndMeth=Nearest  InputSameDT=on
  Relational Operator2 : RelationalOperator  Operator===  OutDataTypeStr=boolean  RndMeth=Nearest  InputSameDT=on
  Switch1 : Switch  Criteria=u2 ~= 0  OutDataTypeStr=Inherit: Inherit via back propagation  SaturateOnIntegerOverflow=on  InputSameDT=on
  Switch2 : Switch  Criteria=u2 ~= 0  OutDataTypeStr=Inherit: Inherit via back propagation  SaturateOnIntegerOverflow=on  InputSameDT=on
  Switch4 : Switch  Criteria=u2 ~= 0  OutDataTypeStr=Inherit: Inherit via back propagation  SaturateOnIntegerOverflow=on  InputSameDT=on
  AFS_dm : Outport
  wires:
  Constant7/1 -> Switch1/1
  Switch2/1 -> Switch1/3
  Relational Operator1/1 -> Switch1/2
  Constant1/1 -> Relational Operator1/1
  Constant5/1 -> Relational Operator1/2
  AFS_facAirSubsEnvPCor_CUR/1 -> Divide/2
  EnvP_p/1 -> AFS_facAirSubsEnvPCor_CUR/1
  DSM_bAFSSysErr/1 -> Logical Operator2/1
  Logical Operator1/1 -> Logical Operator/1
  Logical Operator/1 -> Switch2/2
  Relational Operator/1 -> Logical Operator/2
  Constant3/1 -> Relational Operator/2
  Constant2/1 -> Relational Operator/1
  Divide/1 -> Switch4/1  "AFS_dmSubsVal_mp"
  Epm_nEng/1 -> AFS_dmAirSubsVal_MAP/1
  AFS_dmAirSubsVal_MAP/1 -> Divide/1
  InCtl_qRaw/1 -> AFS_dmAirSubsVal_MAP/2
  ASMod_dmIndAirRef/1 -> Switch4/3
  AFS_dmComp_mp/1 -> Switch2/3
  Switch4/1 -> Switch2/1  "AFS_dmAirSubsVal_mp"
  DSM_bAFS/1 -> Logical Operator1/1
  Switch1/1 -> AFS_dm/1
  Constant4/1 -> Relational Operator2/1
  Constant6/1 -> Relational Operator2/2
  Logical Operator3/1 -> Switch4/2
  Relational Operator2/1 -> Logical Operator3/2
  Logical Operator2/1 -> Logical Operator3/1

== system AFS_VD/AFS_VD/Correction/DriftComp ==
  AFS_dmPlsCorr : Inport
  AFS_dmDrft : Inport  Port=2
  Add1 : Sum  OutDataTypeStr=Inherit: Inherit via back propagation  SaturateOnIntegerOverflow=on  InputSameDT=on
  AFS_dmComp_mp : Outport
  wires:
  AFS_dmDrft/1 -> Add1/2
  Add1/1 -> AFS_dmComp_mp/1
  AFS_dmPlsCorr/1 -> Add1/1

== system AFS_VD/AFS_VD/Correction/Fault_Freeze ==
  note: % If the signal range check for the sensor air mass signal is temporarily erroneous, last valid sensor air mass will be frozen and output %
  AFS_dmSens : Inport
  DSM_bAFSFrzAirMs : Inport  Port=2
  Delay : Delay  DelayLength=1  InitialCondition=0
  Switch1 : Switch  Criteria=u2 ~= 0  OutDataTypeStr=Inherit: Inherit via back propagation  SaturateOnIntegerOverflow=on
  AFS_dmAirFrz_mp : Outport
  wires:
  DSM_bAFSFrzAirMs/1 -> Switch1/2
  AFS_dmSens/1 -> Switch1/1
  Switch1/1 -> Delay/1, AFS_dmAirFrz_mp/1  "AFS_dmAirFrz_mp"
  Delay/1 -> Switch1/3

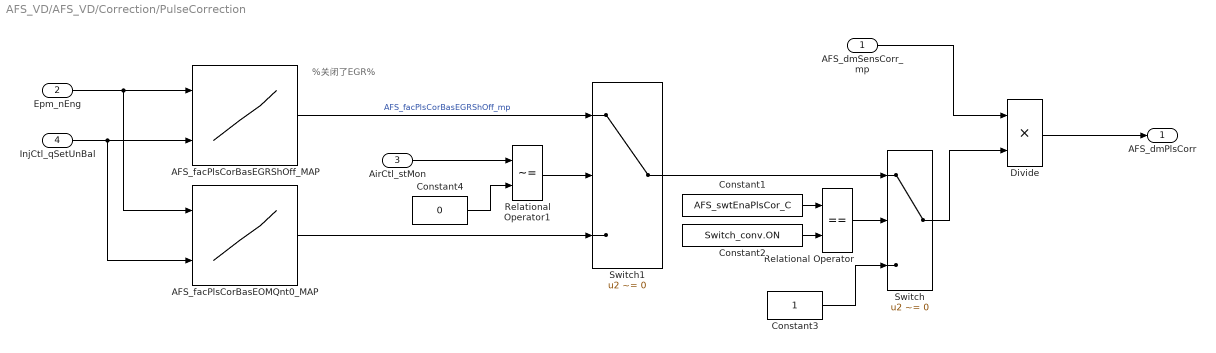
== system AFS_VD/AFS_VD/Correction/PulseCorrection ==
  note: %关闭了EGR%
  AFS_dmSensCorr_mp : Inport
  Epm_nEng : Inport  Port=2
  AirCtl_stMon : Inport  Port=3
  InjCtl_qSetUnBal : Inport  Port=4
  AFS_facPlsCorBasEGRShOff_MAP : Lookup_n-D  BreakpointsForDimension1=AFS_facPlsCorBasEGRShOff_MAPY  BreakpointsForDimension2=AFS_facPlsCorBasEGRShOff_MAPX  IndexSearchMethod=Linear search  BeginIndexSearchUsingPreviousIndexResult=on  Table=AFS_facPlsCorBasEGRShOff_MAP  ExtrapMethod=Clip  UseLastTableValue=on  InternalRulePriority=Speed  OutDataTypeStr=Inherit: Inherit via back propagation  SaturateOnIntegerOverflow=on
  AFS_facPlsCorBasEOMQnt0_MAP : Lookup_n-D  BreakpointsForDimension1=AFS_facPlsCorBasEOMQnt2_MAPY  BreakpointsForDimension2=AFS_facPlsCorBasEOMQnt2_MAPX  IndexSearchMethod=Linear search  BeginIndexSearchUsingPreviousIndexResult=on  Table=AFS_facPlsCorBasEOMQnt2_MAP  ExtrapMethod=Clip  UseLastTableValue=on  InternalRulePriority=Speed  OutDataTypeStr=Inherit: Inherit via back propagation  SaturateOnIntegerOverflow=on
  Constant1 : Constant  Value=AFS_swtEnaPlsCor_C
  Constant2 : Constant  Value=Switch_conv.ON
  Constant3 : Constant  OutDataTypeStr=Inherit: Inherit via back propagation
  Constant4 : Constant  Value=0  OutDataTypeStr=Inherit: Inherit via back propagation
  Divide : Product  Inputs=**  OutDataTypeStr=Inherit: Inherit via back propagation  SaturateOnIntegerOverflow=on
  Relational Operator : RelationalOperator  Operator===  OutDataTypeStr=boolean  RndMeth=Nearest  InputSameDT=on
  Relational Operator1 : RelationalOperator  Operator=~=  OutDataTypeStr=boolean  RndMeth=Nearest  InputSameDT=on
  Switch : Switch  Criteria=u2 ~= 0  OutDataTypeStr=Inherit: Inherit via back propagation  SaturateOnIntegerOverflow=on  InputSameDT=on
  Switch1 : Switch  Criteria=u2 ~= 0  OutDataTypeStr=Inherit: Inherit via back propagation  SaturateOnIntegerOverflow=on  InputSameDT=on
  AFS_dmPlsCorr : Outport
  wires:
  Relational Operator1/1 -> Switch1/2
  Constant4/1 -> Relational Operator1/2
  AirCtl_stMon/1 -> Relational Operator1/1
  Divide/1 -> AFS_dmPlsCorr/1
  Constant3/1 -> Switch/3
  Switch/1 -> Divide/2
  Relational Operator/1 -> Switch/2
  Constant2/1 -> Relational Operator/2
  Constant1/1 -> Relational Operator/1
  Switch1/1 -> Switch/1
  AFS_dmSensCorr_mp/1 -> Divide/1
  Epm_nEng/1 -> AFS_facPlsCorBasEGRShOff_MAP/1, AFS_facPlsCorBasEOMQnt0_MAP/1
  InjCtl_qSetUnBal/1 -> AFS_facPlsCorBasEOMQnt0_MAP/2, AFS_facPlsCorBasEGRShOff_MAP/2
  AFS_facPlsCorBasEGRShOff_MAP/1 -> Switch1/1  "AFS_facPlsCorBasEGRShOff_mp"
  AFS_facPlsCorBasEOMQnt0_MAP/1 -> Switch1/3

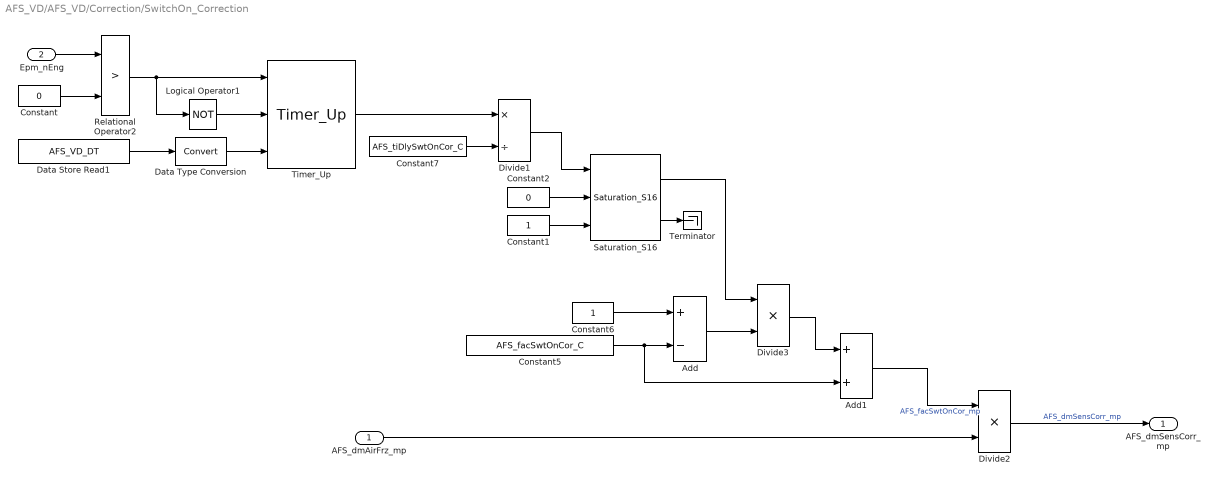
== system AFS_VD/AFS_VD/Correction/SwitchOn_Correction ==
  AFS_dmAirFrz_mp : Inport
  Epm_nEng : Inport  Port=2
  Add : Sum  Inputs=+-  OutDataTypeStr=Inherit: Inherit via back propagation  SaturateOnIntegerOverflow=on  InputSameDT=on
  Add1 : Sum  OutDataTypeStr=Inherit: Inherit via back propagation  SaturateOnIntegerOverflow=on  InputSameDT=on
  Constant : Constant  Value=0  OutDataTypeStr=Inherit: Inherit via back propagation
  Constant1 : Constant  OutDataTypeStr=Inherit: Inherit via back propagation
  Constant2 : Constant  Value=0  OutDataTypeStr=Inherit: Inherit via back propagation
  Constant5 : Constant  Value=AFS_facSwtOnCor_C
  Constant6 : Constant  OutDataTypeStr=Inherit: Inherit via back propagation
  Constant7 : Constant  Value=AFS_tiDlySwtOnCor_C
  Data Store Read1 : DataStoreRead  DataStoreName=AFS_VD_DT
  Data Type Conversion : DataTypeConversion
  Divide1 : Product  Inputs=*/  OutDataTypeStr=Prc_Fact10000  SaturateOnIntegerOverflow=on  InputSameDT=on
  Divide2 : Product  Inputs=**  OutDataTypeStr=Inherit: Inherit via back propagation  SaturateOnIntegerOverflow=on
  Divide3 : Product  Inputs=**  OutDataTypeStr=Inherit: Inherit via back propagation  SaturateOnIntegerOverflow=on
  Logical Operator1 : Logic  Operator=NOT  AllPortsSameDT=off  OutDataTypeStr=boolean
  Relational Operator2 : RelationalOperator  Operator=>  OutDataTypeStr=boolean  RndMeth=Nearest  InputSameDT=on
  Saturation_S16 : CXLib/Saturation_S16
  Terminator : Terminator
  Timer_Up : CXLib/Timer_Up
  AFS_dmSensCorr_mp : Outport
  wires:
  Divide2/1 -> AFS_dmSensCorr_mp/1  "AFS_dmSensCorr_mp"
  Constant5/1 -> Add/2, Add1/2
  Divide3/1 -> Add1/1
  Constant7/1 -> Divide1/2
  Constant6/1 -> Add/1
  Relational Operator2/1 -> Timer_Up/1, Logical Operator1/1
  Constant/1 -> Relational Operator2/2
  Data Store Read1/1 -> Data Type Conversion/1
  Timer_Up/1 -> Divide1/1
  Logical Operator1/1 -> Timer_Up/2
  Epm_nEng/1 -> Relational Operator2/1
  Constant1/1 -> Saturation_S16/3
  Constant2/1 -> Saturation_S16/2
  Divide1/1 -> Saturation_S16/1
  Saturation_S16/2 -> Terminator/1
  Saturation_S16/1 -> Divide3/1
  Add/1 -> Divide3/2
  Add1/1 -> Divide2/1  "AFS_facSwtOnCor_mp"
  AFS_dmAirFrz_mp/1 -> Divide2/2
  Data Type Conversion/1 -> Timer_Up/3

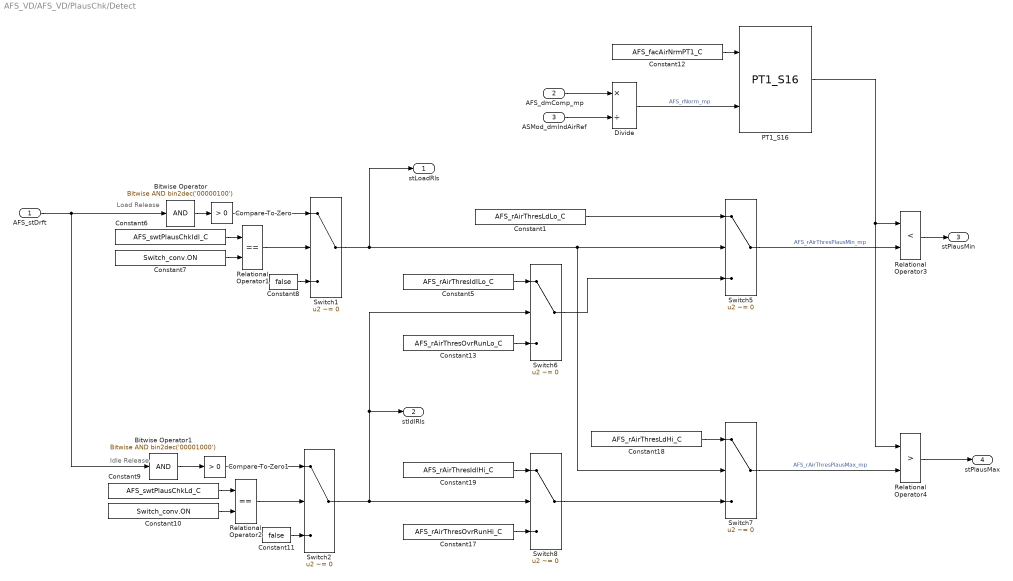
== system AFS_VD/AFS_VD/PlausChk/Detect ==
  note: Load Release
  note: Idle Release
  AFS_stDrft : Inport
  AFS_dmComp_mp : Inport  Port=2
  ASMod_dmIndAirRef : Inport  Port=3
  Bitwise Operator : simulink/Logic and Bit Operations/Bitwise Operator  logicop=AND  UseBitMask=on  BitMask=bin2dec('00000100')  BitMaskRealWorld=Stored Integer
  Bitwise Operator1 : simulink/Logic and Bit Operations/Bitwise Operator  logicop=AND  UseBitMask=on  BitMask=bin2dec('00001000')  BitMaskRealWorld=Stored Integer
  Compare To Zero : simulink/Logic and Bit Operations/Compare To Zero  relop=>  OutDataTypeStr=boolean
  Compare To Zero1 : simulink/Logic and Bit Operations/Compare To Zero  relop=>  OutDataTypeStr=boolean
  Constant1 : Constant  Value=AFS_rAirThresLdLo_C
  Constant10 : Constant  Value=Switch_conv.ON
  Constant11 : Constant  Value=false  OutDataTypeStr=Inherit: Inherit via back propagation
  Constant12 : Constant  Value=AFS_facAirNrmPT1_C
  Constant13 : Constant  Value=AFS_rAirThresOvrRunLo_C
  Constant17 : Constant  Value=AFS_rAirThresOvrRunHi_C
  Constant18 : Constant  Value=AFS_rAirThresLdHi_C
  Constant19 : Constant  Value=AFS_rAirThresIdlHi_C
  Constant5 : Constant  Value=AFS_rAirThresIdlLo_C
  Constant6 : Constant  Value=AFS_swtPlausChkIdl_C
  Constant7 : Constant  Value=Switch_conv.ON
  Constant8 : Constant  Value=false  OutDataTypeStr=Inherit: Inherit via back propagation
  Constant9 : Constant  Value=AFS_swtPlausChkLd_C
  Divide : Product  Inputs=*/  OutDataTypeStr=Inherit: Inherit via back propagation  SaturateOnIntegerOverflow=on
  PT1_S16 : CXLib/PT1_S16
  Relational Operator1 : RelationalOperator  Operator===  OutDataTypeStr=boolean  RndMeth=Nearest  InputSameDT=on
  Relational Operator2 : RelationalOperator  Operator===  OutDataTypeStr=boolean  RndMeth=Nearest  InputSameDT=on
  Relational Operator3 : RelationalOperator  Operator=<  OutDataTypeStr=boolean  RndMeth=Simplest  InputSameDT=on
  Relational Operator4 : RelationalOperator  Operator=>  OutDataTypeStr=boolean  RndMeth=Simplest  InputSameDT=on
  Switch{1..2,5..8} (6 alike) : Switch  Criteria=u2 ~= 0  OutDataTypeStr=Inherit: Inherit via back propagation  SaturateOnIntegerOverflow=on  InputSameDT=on
  stLoadRls : Outport
  stIdlRls : Outport  Port=2
  stPlausMin : Outport  Port=3
  stPlausMax : Outport  Port=4
  wires:
  Switch8/1 -> Switch7/3
  Constant13/1 -> Switch6/3
  Constant5/1 -> Switch6/1
  Switch6/1 -> Switch5/3
  Constant1/1 -> Switch5/1
  Compare To Zero1/1 -> Switch2/1
  Bitwise Operator1/1 -> Compare To Zero1/1
  Compare To Zero/1 -> Switch1/1
  Bitwise Operator/1 -> Compare To Zero/1
  Relational Operator4/1 -> stPlausMax/1
  Relational Operator3/1 -> stPlausMin/1
  PT1_S16/1 -> Relational Operator4/1, Relational Operator3/1
  Switch2/1 -> Switch6/2, stIdlRls/1, Switch8/2
  Divide/1 -> PT1_S16/2  "AFS_rNorm_mp"
  AFS_dmComp_mp/1 -> Divide/1
  ASMod_dmIndAirRef/1 -> Divide/2
  Constant12/1 -> PT1_S16/1
  AFS_stDrft/1 -> Bitwise Operator1/1, Bitwise Operator/1
  Constant11/1 -> Switch2/3
  Relational Operator2/1 -> Switch2/2
  Constant10/1 -> Relational Operator2/2
  Constant9/1 -> Relational Operator2/1
  Switch1/1 -> stLoadRls/1, Switch7/2, Switch5/2
  Constant7/1 -> Relational Operator1/2
  Constant8/1 -> Switch1/3
  Relational Operator1/1 -> Switch1/2
  Constant6/1 -> Relational Operator1/1
  Constant17/1 -> Switch8/3
  Constant19/1 -> Switch8/1
  Constant18/1 -> Switch7/1
  Switch7/1 -> Relational Operator4/2  "AFS_rAirThresPlausMax_mp"
  Switch5/1 -> Relational Operator3/2  "AFS_rAirThresPlausMin_mp"

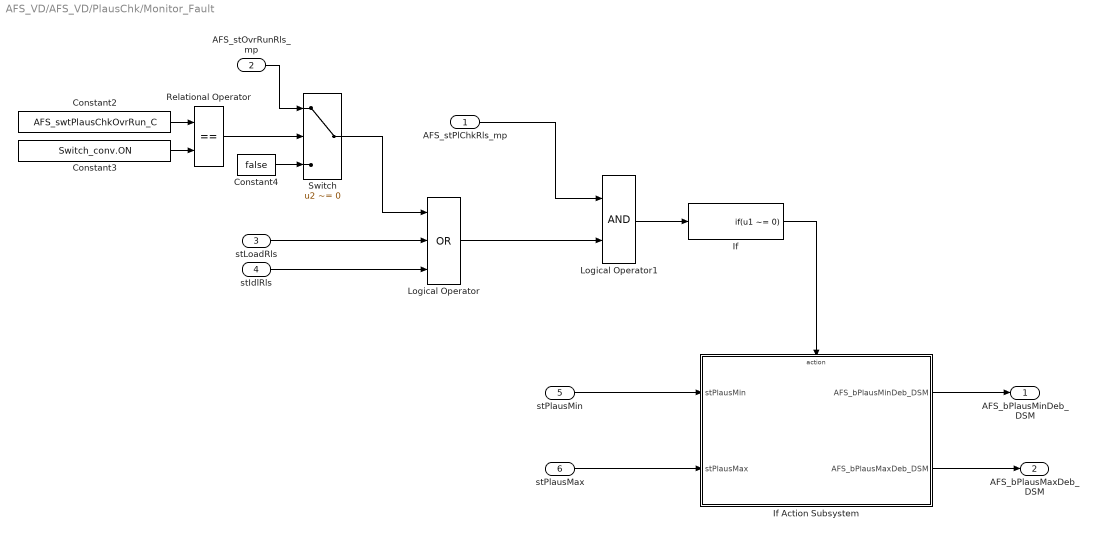
== system AFS_VD/AFS_VD/PlausChk/Monitor_Fault ==
  AFS_stPlChkRls_mp : Inport
  AFS_stOvrRunRls_mp : Inport  Port=2
  stLoadRls : Inport  Port=3
  stIdlRls : Inport  Port=4
  stPlausMin : Inport  Port=5
  stPlausMax : Inport  Port=6
  Constant2 : Constant  Value=AFS_swtPlausChkOvrRun_C
  Constant3 : Constant  Value=Switch_conv.ON
  Constant4 : Constant  Value=false  OutDataTypeStr=Inherit: Inherit via back propagation
  If : If  IfExpression=u1 ~= 0  ShowElse=off
  If Action Subsystem : Subsystem  TreatAsAtomicUnit=on
  Logical Operator : Logic  Operator=OR  Inputs=3  OutDataTypeStr=boolean
  Logical Operator1 : Logic  OutDataTypeStr=boolean
  Relational Operator : RelationalOperator  Operator===  OutDataTypeStr=boolean  RndMeth=Nearest  InputSameDT=on
  Switch : Switch  Criteria=u2 ~= 0  OutDataTypeStr=Inherit: Inherit via back propagation  SaturateOnIntegerOverflow=on  InputSameDT=on
  AFS_bPlausMinDeb_DSM : Outport
  AFS_bPlausMaxDeb_DSM : Outport  Port=2
  wires:
  Switch/1 -> Logical Operator/1
  Constant4/1 -> Switch/3
  AFS_stOvrRunRls_mp/1 -> Switch/1
  AFS_stPlChkRls_mp/1 -> Logical Operator1/1
  Logical Operator/1 -> Logical Operator1/2
  Logical Operator1/1 -> If/1
  Constant2/1 -> Relational Operator/1
  Relational Operator/1 -> Switch/2
  Constant3/1 -> Relational Operator/2
  stLoadRls/1 -> Logical Operator/2
  stIdlRls/1 -> Logical Operator/3
  stPlausMin/1 -> If Action Subsystem/1(stPlausMin)
  stPlausMax/1 -> If Action Subsystem/2(stPlausMax)
  If Action Subsystem/1(AFS_bPlausMinDeb_DSM) -> AFS_bPlausMinDeb_DSM/1
  If Action Subsystem/2(AFS_bPlausMaxDeb_DSM) -> AFS_bPlausMaxDeb_DSM/1
  If/1 -> If Action Subsystem/Action

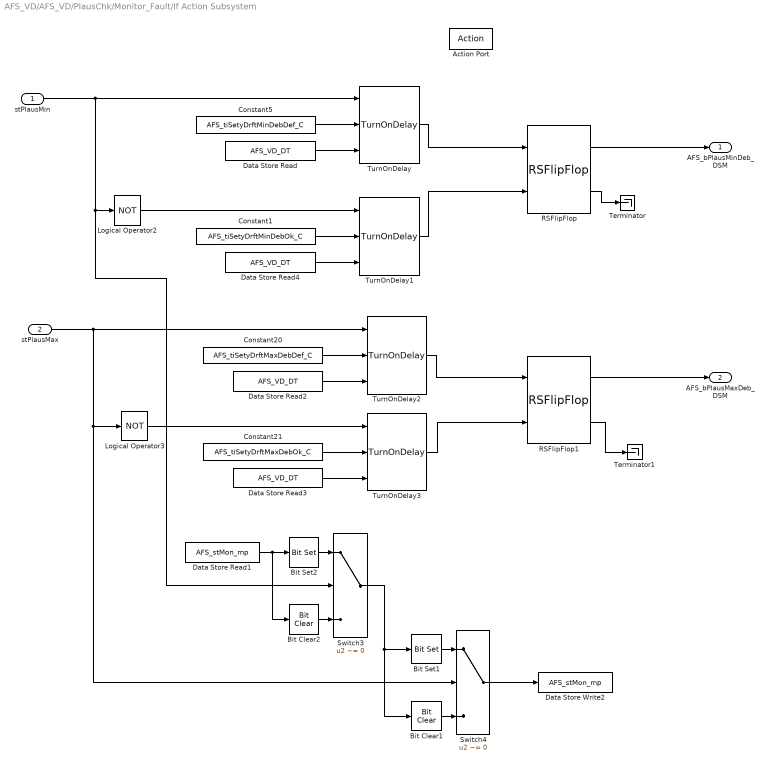
== system AFS_VD/AFS_VD/PlausChk/Monitor_Fault/If Action Subsystem ==
  stPlausMin : Inport
  stPlausMax : Inport  Port=2
  Action Port : ActionPort  ActionType=then
  Bit Clear1 : simulink/Logic and Bit Operations/Bit Clear  iBit=26
  Bit Clear2 : simulink/Logic and Bit Operations/Bit Clear  iBit=25
  Bit Set1 : simulink/Logic and Bit Operations/Bit Set  iBit=26
  Bit Set2 : simulink/Logic and Bit Operations/Bit Set  iBit=25
  Constant1 : Constant  Value=AFS_tiSetyDrftMinDebOk_C
  Constant20 : Constant  Value=AFS_tiSetyDrftMaxDebDef_C
  Constant21 : Constant  Value=AFS_tiSetyDrftMaxDebOk_C
  Constant5 : Constant  Value=AFS_tiSetyDrftMinDebDef_C
  Data Store Read{,2..4} (4 alike) : DataStoreRead  DataStoreName=AFS_VD_DT
  Data Store Read1 : DataStoreRead  DataStoreName=AFS_stMon_mp
  Data Store Write2 : DataStoreWrite  DataStoreName=AFS_stMon_mp
  Logical Operator2 : Logic  Operator=NOT  AllPortsSameDT=off  OutDataTypeStr=boolean
  Logical Operator3 : Logic  Operator=NOT  AllPortsSameDT=off  OutDataTypeStr=boolean
  RSFlipFlop : CXLib/RSFlipFlop
  RSFlipFlop1 : CXLib/RSFlipFlop
  Switch3 : Switch  Criteria=u2 ~= 0  OutDataTypeStr=Inherit: Inherit via back propagation  SaturateOnIntegerOverflow=on  InputSameDT=on
  Switch4 : Switch  Criteria=u2 ~= 0  OutDataTypeStr=Inherit: Inherit via back propagation  SaturateOnIntegerOverflow=on  InputSameDT=on
  Terminator : Terminator
  Terminator1 : Terminator
  TurnOnDelay{,1..3} (4 alike) : CXLib/TurnOnDelay
  AFS_bPlausMinDeb_DSM : Outport
  AFS_bPlausMaxDeb_DSM : Outport  Port=2
  wires:
  Data Store Read3/1 -> TurnOnDelay3/3
  Data Store Read2/1 -> TurnOnDelay2/3
  Data Store Read4/1 -> TurnOnDelay1/3
  Data Store Read/1 -> TurnOnDelay/3
  stPlausMin/1 -> TurnOnDelay/1, Switch3/2, Logical Operator2/1
  RSFlipFlop1/2 -> Terminator1/1
  RSFlipFlop/2 -> Terminator/1
  Constant21/1 -> TurnOnDelay3/2
  TurnOnDelay3/1 -> RSFlipFlop1/2
  Logical Operator3/1 -> TurnOnDelay3/1
  TurnOnDelay2/1 -> RSFlipFlop1/1
  Logical Operator2/1 -> TurnOnDelay1/1
  TurnOnDelay/1 -> RSFlipFlop/1
  Constant5/1 -> TurnOnDelay/2
  Constant1/1 -> TurnOnDelay1/2
  Constant20/1 -> TurnOnDelay2/2
  TurnOnDelay1/1 -> RSFlipFlop/2
  Switch4/1 -> Data Store Write2/1
  Switch3/1 -> Bit Set1/1, Bit Clear1/1
  Bit Set1/1 -> Switch4/1
  Bit Clear1/1 -> Switch4/3
  Data Store Read1/1 -> Bit Set2/1, Bit Clear2/1
  Bit Set2/1 -> Switch3/1
  Bit Clear2/1 -> Switch3/3
  RSFlipFlop/1 -> AFS_bPlausMinDeb_DSM/1
  RSFlipFlop1/1 -> AFS_bPlausMaxDeb_DSM/1
  stPlausMax/1 -> Switch4/2, Logical Operator3/1, TurnOnDelay2/1
